simulink model "Lateral_control"  (R2022a)
settings: Solver=VariableStepAuto  StartTime=0.0  StopTime=15  RelTol=1e-3
values from neighbouring files (symbols this model uses):
  Cf = 19000    [main.m]
  Cr = 33000    [main.m]
  Iz = 2875    [main.m]
  Kfb = K(1,1:end-2)    [main.m]
  Kff = K(1,5:end)    [main.m]
  Lf = 1.2    [main.m]
  Lr = 1.6    [main.m]
  m = 1575    [main.m]
  Vx = 10    [main.m]
  x_0 = [0 0 0 0]'    [main.m]
undefined symbols (not defined in the file or in its folder): driving, sigbuilder_block
libraries: drivingscenarioandsensors x2
settings Model: Creator=User  LastModifiedBy=User

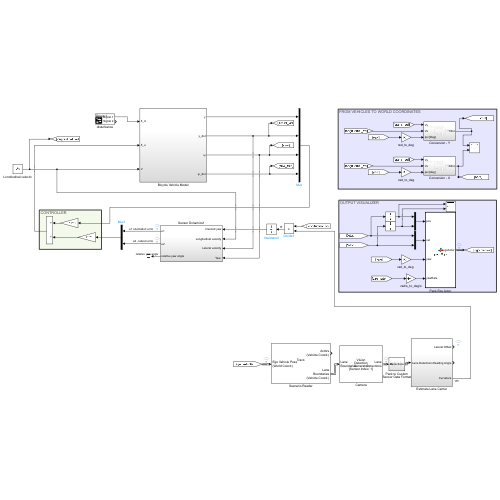
[thumbnail: Simulink's stored preview of the top-level diagram]
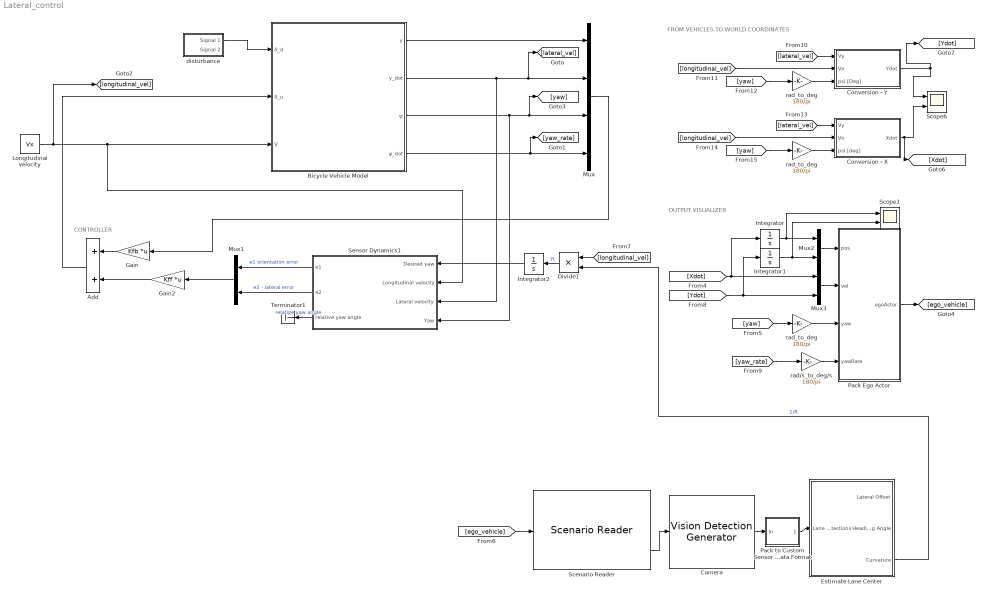
== system Lateral_control ==
  note: CONTROLLER
  note: FROM VEHICLES TO WORLD COORDINATES
  note: OUTPUT VISUALIZER
  Add : Sum
  Bicycle Vehicle Model : Subsystem
  Camera : drivingscenarioandsensors/Vision Detection Generator  SensorIndex=1  DetectorOutput=Lanes only  UpdateInterval=0.01  LaneUpdateInterval=0.01  SensorLocation=[1.9 0]  Height=1.1  Yaw=0  Pitch=1  Roll=0  BusNameSource=Auto  BusName=BusObjectDetections  BusName2Source=Property  BusName2=BusVision  MaxNumDetectionsSource=Property  MaxNumDetections=50  MaxNumLanesSource=Property  MaxNumLanes=2  DetectionCoordinates=Ego Cartesian  SimulateUsing=Interpreted execution  MaxRange=150  BoundingBoxAccuracy=5  ProcessNoiseIntensity=5  MaxSpeed=50  MaxAllowedOcclusion=0.5  MinObjectImageSize=[15 15]  DetectionProbability=0.9  FalsePositivesPerImage=0.1  MinLaneImageSize=[20 3]  LaneBoundaryAccuracy=3  HasNoise=on  InitialSeedSource=Repeatable  InitialSeed=0  UsedSeed=0  ActorProfilesSource=Parameters  ActorProfilesParameters=driving.internal.ActorProfilesParameters  ActorProfilesExpression=[struct('ActorID',1,'ClassID',1,'Length',4.7,'Width',1.8,'Height',1.4,'OriginOffset',[-1.35 0 0],'MeshVertices',[3.7 -0.9 1.4;3.7 0.9 1.4;-1 0.9 1.4;-1 -0.9 1.4;3.7 -0.9 0;3.7 0.9 0;-1 0.9 0;-1 -0.9 0],'MeshFaces',[6 2 1;1 5 6;8 4 3;3 7 8;6 7 3;3 2 6;5 1 4;4 8 5;4 1 2;2 3 4;7 6 5;5 8 7],'RCSPattern',[10 10;10 10],'RCSAzimuthAngles',[-180 180],'RCSElevationAngles',[-90 90])]  Intrinsics=driving.internal.cameraIntrinsics('FocalLength',[800 800],'PrincipalPoint',[320 240],'ImageSize',[480 640],'RadialDistortion',[0 0],'TangentialDistortion',[0 0],'Skew',0)
  Conversion - X : Subsystem
  Conversion - Y : Subsystem
  Divide1 : Product  Inputs=**
  Estimate Lane Center : Subsystem  VariantControl=v2
  Gain : Gain  Gain=Kfb  Multiplication=Matrix(K*u)
  Gain2 : Gain  Gain=Kff  Multiplication=Matrix(K*u)
  Integrator : Integrator  InitialCondition=1.64
  Integrator1 : Integrator  InitialCondition=0.05
  Integrator2 : Integrator
  Longitudinal velocity : Constant  Value=Vx  SampleTime=-1
  Mux : Mux
  Mux1 : Mux  Inputs=2
  Mux2 : Mux  Inputs=2
  Mux3 : Mux  Inputs=2
  Pack Ego Actor : MATLAB Function  TreatAsAtomicUnit=on
  Pack to Custom Sensor Data Format : Subsystem
  Scenario Reader : drivingscenarioandsensors/Scenario Reader  ScenarioSource=From file  ScenarioFileName=Track.mat  ScenarioVariableName=scenario  OutputCoordinateSystem=Vehicle coordinates  EgoVehicleSource=Input port  EgoVehicleActorID=1  OrientVehiclesOnRoad=off  OutputEgoVehiclePose=off  OutputEgoVehicleState=off  SampleTime=0.01  LaneBoundaryOutput=Ego vehicle lane boundaries  LaneBoundaryDistance=linspace(-150, 150, 101)  LaneBoundaryLocation=Center of lane markings  BusNameSource=Auto  BusName=BusActors  BusNumActorsSource=Scenario  BusNumActors=100  BusName2Source=Auto  BusName2=BusLaneBoundaries  BusNumLaneBoundariesSource=Scenario  BusNumLaneBoundaries=10  BusName3Source=Auto  BusName3=BusEgoActor  BusName4Source=Auto  BusName4=BusEgoState  ShowCoordinateLabels=on  SimulateUsing=Interpreted execution
  Scope1 : Scope  NumInputPorts=2
  Scope6 : Scope  NumInputPorts=2
  Sensor Dynamics1 : Subsystem
  Terminator1 : Terminator
  disturbance : Subsystem  Tag=STV Subsys  LoadFcn=sigbuilder_block('load');  StartFcn=sigbuilder_block('start');  StopFcn=sigbuilder_block('stop');  ClipboardFcn=sigbuilder_block('clipboard');  mask(Sigbuilder block){tuvar=[0:10]}
      mask help: Simulink:masks:SigbuilderBlock_MD
      mask init:
      | if ~strcmp(get_param(bdroot(gcbh),'SimulationStatus'),'stopped') tuvar = sigbuilder_block('maskInit'); end
      settings: CopyFcn=sigbuilder_block('copy');  DeleteFcn=sigbuilder_block('delete');  ModelCloseFcn=sigbuilder_block('modelClose');  PreSaveFcn=sigbuilder_block('preSave');  PauseFcn=sigbuilder_block('pause');  ContinueFcn=sigbuilder_block('continue');  NameChangeFcn=sigbuilder_block('namechange');  OpenFcn=sigbuilder_block('open',[5.4 44.4 1141.2 541.8 ]);  CloseFcn=sigbuilder_block('close');
      mask Display: plot(0, 0, 100, 100,[2, 2, 32, 32, 2], [68, 8, 8, 68, 68],[32, 2], [38, 38], [32, 19, 2],[53, 60, 44], [32, 17, 17, 2],[16, 16, 31, 31]);txt = getActiveGroup(gcbh);text(2, 100, txt,'verticalAlignment', 'top');
  rad/s_to_deg/s : Gain  Gain=180/pi
  rad_to_deg : Gain  Gain=180/pi
  "rad_to_deg " : Gain  Gain=180/pi
  "rad_to_deg  " : Gain  Gain=180/pi
  wires:
  Add/1 -> Bicycle Vehicle Model/2(δ_u)
  rad_to_deg/1 -> Conversion - X/3(psi [deg])
  [longitudinal_vel] -> Conversion - X/2(Vx)
  Bicycle Vehicle Model/4(ψ_dot) -> [yaw_rate], Mux/4
  Pack to Custom Sensor Data Format/1(Lane Detections) -> Estimate Lane Center/1(Lane Detections)
  Conversion - Y/1(Ydot) -> [Ydot], Scope6/1
  Divide1/1 -> Integrator2/1  "R"
  "rad_to_deg "/1 -> Conversion - Y/3(psi [Deg])
  Integrator/1 -> Scope1/1, Mux2/1
  rad/s_to_deg/s/1 -> Pack Ego Actor/4(yawRate)
  Mux1/1 -> Gain2/1
  [lateral_vel] -> Conversion - X/1(Vy)
  Integrator1/1 -> Scope1/2, Mux2/2
  Gain2/1 -> Add/2
  Mux2/1 -> Pack Ego Actor/1(pos)
  Mux3/1 -> Pack Ego Actor/2(vel)
  [yaw_rate] -> rad/s_to_deg/s/1
  Bicycle Vehicle Model/2(y_dot) -> Sensor Dynamics1/3(Lateral velocity), [lateral_vel], Mux/2
  "rad_to_deg  "/1 -> Pack Ego Actor/3(yaw)
  Sensor Dynamics1/1(e1) -> Mux1/1  "e1 orientation error"
  Camera/1 -> Pack to Custom Sensor Data Format/1(In)
  [yaw] -> "rad_to_deg  "/1
  Conversion - X/1(Xdot) -> Scope6/2, [Xdot]
  Sensor Dynamics1/2(e2) -> Mux1/2  "e2 - lateral error"
  Sensor Dynamics1/3(relative yaw angle) -> Terminator1/1  "relative yaw angle"
  Integrator2/1 -> Sensor Dynamics1/1(Desired yaw)
  [Ydot] -> Integrator1/1, Mux3/2
  [Xdot] -> Integrator/1, Mux3/1
  [yaw] -> "rad_to_deg "/1
  [ego_vehicle] -> Scenario Reader/1
  [longitudinal_vel] -> Conversion - Y/2(Vx)
  [longitudinal_vel] -> Divide1/1
  Pack Ego Actor/1(egoActor) -> [ego_vehicle]
  [lateral_vel] -> Conversion - Y/1(Vy)
  Bicycle Vehicle Model/3(ψ) -> Sensor Dynamics1/4("Yaw "), [yaw], Mux/3
  Gain/1 -> Add/1
  [yaw] -> rad_to_deg/1
  Scenario Reader/2 -> Camera/1
  Bicycle Vehicle Model/1(y) -> Mux/1
  Mux/1 -> Gain/1
  Longitudinal velocity/1 -> Sensor Dynamics1/2(Longitudinal velocity), Bicycle Vehicle Model/3(V), [longitudinal_vel]
  Estimate Lane Center/3(Curvature) -> Divide1/2  "1/R"
  disturbance/1(Signal 1) -> Bicycle Vehicle Model/1(δ_d)

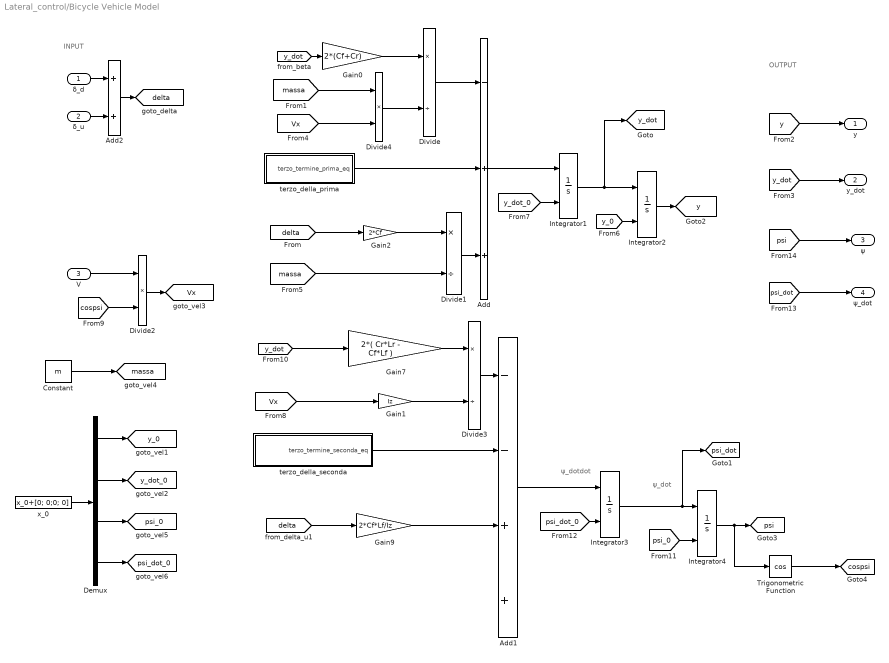
== system Lateral_control/Bicycle Vehicle Model ==
  note: ψ_dot
  note: OUTPUT
  note: INPUT
  note: ψ_dotdot
  δ_d : Inport
  δ_u : Inport  Port=2
  V : Inport  Port=3
  Add : Sum  Inputs=-++
  Add1 : Sum  Inputs=--++
  Add2 : Sum
  Constant : Constant  Value=m
  Demux : Demux
  Divide : Product  Inputs=*/
  Divide1 : Product  Inputs=*/
  Divide2 : Product  Inputs=**
  Divide3 : Product  Inputs=*/
  Divide4 : Product  Inputs=**
  Gain0 : Gain  Gain=2*(Cf+Cr)
  Gain1 : Gain  Gain=Iz
  Gain2 : Gain  Gain=2*Cf
  Gain7 : Gain  Gain="2*( Cr*Lr  - Cf*Lf )"
  Gain9 : Gain  Gain=2*Cf*Lf/Iz
  Integrator1 : Integrator  InitialConditionSource=external
  Integrator2 : Integrator  InitialConditionSource=external
  Integrator3 : Integrator  InitialConditionSource=external
  Integrator4 : Integrator  InitialConditionSource=external  LowerSaturationLimit=0
  Trigonometric Function : Trigonometry  Operator=cos
  terzo_della_prima : Subsystem
  terzo_della_seconda : Subsystem
  "x_0 " : Constant  Value=x_0+[0; 0;0; 0]
  y : Outport
  y_dot : Outport  Port=2
  ψ : Outport  Port=3
  ψ_dot : Outport  Port=4
  tag scope: Vx=global, cospsi=global, delta=global, massa=global, psi=global, psi_0=global, psi_dot=global, psi_dot_0=global, y=global, y_0=global, y_dot=global, y_dot_0=global
  wires:
  [psi] -> ψ/1
  [psi_dot] -> ψ_dot/1
  [psi_dot_0] -> Integrator3/2
  [psi_0] -> Integrator4/2
  [cospsi] -> Divide2/2
  Trigonometric Function/1 -> [cospsi]
  Divide2/1 -> [Vx]
  Integrator4/1 -> [psi], Trigonometric Function/1
  [Vx] -> Gain1/1
  Gain1/1 -> Divide3/2
  Divide3/1 -> Add1/1
  [y_0] -> Integrator2/2
  [y_dot_0] -> Integrator1/2
  Demux/4 -> [psi_dot_0]
  Demux/3 -> [psi_0]
  Integrator2/1 -> [y]
  Integrator1/1 -> [y_dot], Integrator2/1
  Divide1/1 -> Add/3
  [massa] -> Divide1/2
  Divide/1 -> Add/1
  [Vx] -> Divide4/2
  [massa] -> Divide4/1
  Divide4/1 -> Divide/2
  "x_0 "/1 -> Demux/1
  [delta] -> Gain2/1
  Add2/1 -> [delta]
  Gain9/1 -> Add1/3
  terzo_della_seconda/1("terzo_termine_seconda_eq ") -> Add1/2
  Gain2/1 -> Divide1/1
  terzo_della_prima/1("terzo_termine_prima_eq ") -> Add/2
  Demux/2 -> [y_dot_0]
  Demux/1 -> [y_0]
  Constant/1 -> [massa]
  Integrator3/1 -> Integrator4/1, [psi_dot]
  Add/1 -> Integrator1/1
  [y_dot] -> Gain7/1
  [y_dot] -> Gain0/1
  [y_dot] -> y_dot/1
  [y] -> y/1
  [delta] -> Gain9/1
  Gain7/1 -> Divide3/1
  Add1/1 -> Integrator3/1
  Gain0/1 -> Divide/1
  V/1 -> Divide2/1
  δ_u/1 -> Add2/2
  δ_d/1 -> Add2/1

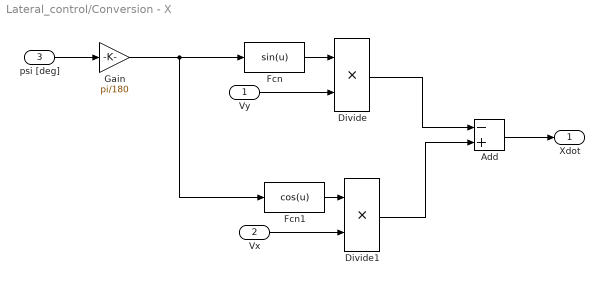
== system Lateral_control/Conversion - X ==
  Vy : Inport
  Vx : Inport  Port=2
  psi [deg] : Inport  Port=3
  Add : Sum  Inputs=-+
  Divide : Product  Inputs=**
  Divide1 : Product  Inputs=**
  Fcn : Fcn  Expr=sin(u)
  Fcn1 : Fcn  Expr=cos(u)
  Gain : Gain  Gain=pi/180
  Xdot : Outport
  wires:
  Gain/1 -> Fcn/1, Fcn1/1
  Add/1 -> Xdot/1
  Divide1/1 -> Add/2
  Vx/1 -> Divide1/2
  Fcn1/1 -> Divide1/1
  Divide/1 -> Add/1
  Vy/1 -> Divide/2
  Fcn/1 -> Divide/1
  psi [deg]/1 -> Gain/1

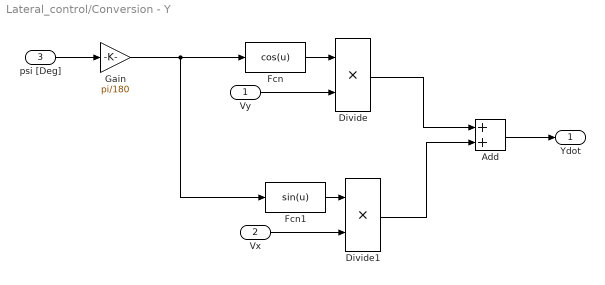
== system Lateral_control/Conversion - Y ==
  Vy : Inport
  Vx : Inport  Port=2
  psi [Deg] : Inport  Port=3
  Add : Sum
  Divide : Product  Inputs=**
  Divide1 : Product  Inputs=**
  Fcn : Fcn  Expr=cos(u)
  Fcn1 : Fcn  Expr=sin(u)
  Gain : Gain  Gain=pi/180
  Ydot : Outport
  wires:
  psi [Deg]/1 -> Gain/1
  Fcn/1 -> Divide/1
  Vy/1 -> Divide/2
  Divide/1 -> Add/1
  Fcn1/1 -> Divide1/1
  Vx/1 -> Divide1/2
  Divide1/1 -> Add/2
  Add/1 -> Ydot/1
  Gain/1 -> Fcn1/1, Fcn/1

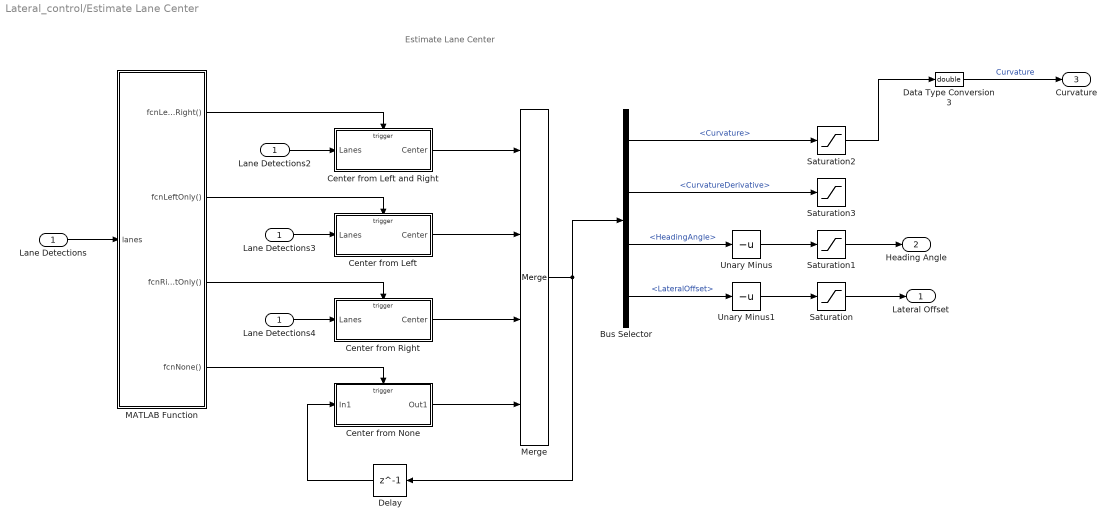
== system Lateral_control/Estimate Lane Center ==
  note: Estimate Lane Center
  Lane Detections : Inport
  Bus Selector : BusSelector  OutputSignals=Curvature,CurvatureDerivative,HeadingAngle,LateralOffset
  Center from Left : Subsystem  TreatAsAtomicUnit=on
  Center from Left and Right : Subsystem  TreatAsAtomicUnit=on
  Center from None : Subsystem  TreatAsAtomicUnit=on
  Center from Right : Subsystem  TreatAsAtomicUnit=on
  Data Type Conversion3 : DataTypeConversion  OutDataTypeStr=double  SaturateOnIntegerOverflow=off  RndMeth=Floor
  Delay : Delay  DelayLength=1
  Lane Detections2 : InportShadow
  Lane Detections3 : InportShadow
  Lane Detections4 : InportShadow
  MATLAB Function : MATLAB Function  TreatAsAtomicUnit=on
  Merge : Merge  Inputs=4
  Saturation : Saturate
  Saturation1 : Saturate  UpperLimit=0.6  LowerLimit=-0.6
  Saturation2 : Saturate  UpperLimit=0.15  LowerLimit=-0.15
  Saturation3 : Saturate  UpperLimit=0.15  LowerLimit=-0.15
  Unary Minus : UnaryMinus
  Unary Minus1 : UnaryMinus
  Lateral Offset : Outport  VectorParamsAs1DForOutWhenUnconnected=off
  Heading Angle : Outport  Port=2  VectorParamsAs1DForOutWhenUnconnected=off
  Curvature : Outport  Port=3  VectorParamsAs1DForOutWhenUnconnected=off
  wires:
  Center from Right/1(Center) -> Merge/3
  Lane Detections3/1 -> Center from Left/1(Lanes)
  Lane Detections4/1 -> Center from Right/1(Lanes)
  MATLAB Function/2(fcnLeftOnly()) -> Center from Left/Trigger
  Center from None/1(Out1) -> Merge/4
  MATLAB Function/1(fcnLeftAndRight()) -> Center from Left and Right/Trigger
  Delay/1 -> Center from None/1(In1)
  Center from Left and Right/1(Center) -> Merge/1
  Lane Detections/1 -> MATLAB Function/1(lanes)
  Lane Detections2/1 -> Center from Left and Right/1(Lanes)
  MATLAB Function/3(fcnRightOnly()) -> Center from Right/Trigger
  MATLAB Function/4(fcnNone()) -> Center from None/Trigger
  Center from Left/1(Center) -> Merge/2
  Merge/1 -> Bus Selector/1, Delay/1
  Saturation2/1 -> Data Type Conversion3/1
  Saturation1/1 -> Heading Angle/1
  Saturation/1 -> Lateral Offset/1
  Unary Minus/1 -> Saturation1/1
  Bus Selector/2 -> Saturation3/1  "<CurvatureDerivative>"
  Bus Selector/1 -> Saturation2/1  "<Curvature>"
  Unary Minus1/1 -> Saturation/1
  Bus Selector/4 -> Unary Minus1/1  "<LateralOffset>"
  Bus Selector/3 -> Unary Minus/1  "<HeadingAngle>"
  Data Type Conversion3/1 -> Curvature/1  "Curvature"

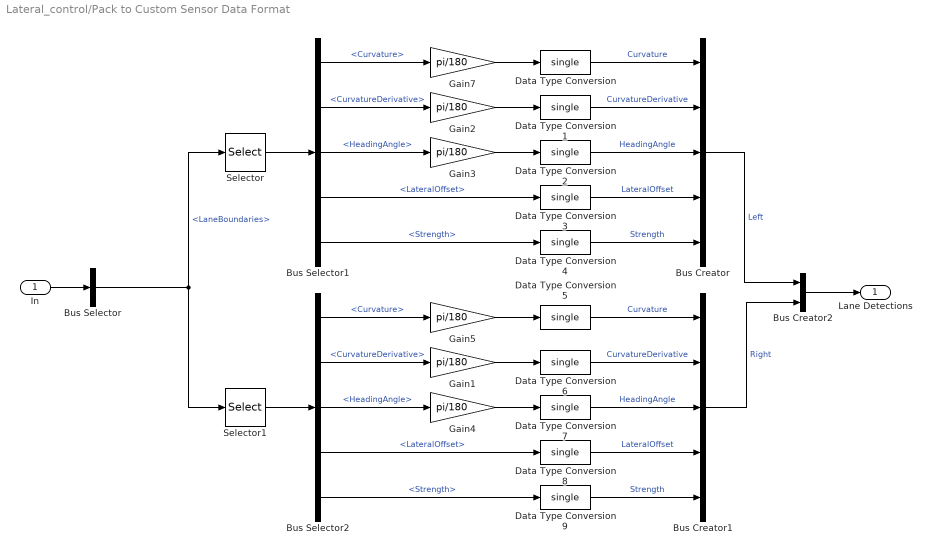
== system Lateral_control/Pack to Custom Sensor Data Format ==
  In : Inport
  Bus Creator : BusCreator  Inputs=5  OutDataTypeStr=Bus: LaneSensorBoundaries
  Bus Creator1 : BusCreator  Inputs=5  OutDataTypeStr=Bus: LaneSensorBoundaries
  Bus Creator2 : BusCreator  Inputs=2  OutDataTypeStr=Bus: LaneSensor
  Bus Selector : BusSelector  OutputSignals=LaneBoundaries
  Bus Selector1 : BusSelector  OutputSignals=Curvature,CurvatureDerivative,HeadingAngle,LateralOffset,Strength
  Bus Selector2 : BusSelector  OutputSignals=Curvature,CurvatureDerivative,HeadingAngle,LateralOffset,Strength
  Data Type Conversion{,1..9} (10 alike) : DataTypeConversion  OutDataTypeStr=single  SaturateOnIntegerOverflow=off  RndMeth=Floor
  Gain{1..5,7} (6 alike) : Gain  Gain=pi/180
  Selector : Selector  InputPortWidth=2  IndexOptions=Index vector (dialog)  Indices=1  OutputSizes=1
  Selector1 : Selector  InputPortWidth=2  IndexOptions=Index vector (dialog)  Indices=2  OutputSizes=1
  Lane Detections : Outport  VectorParamsAs1DForOutWhenUnconnected=off
  wires:
  In/1 -> Bus Selector/1
  Bus Selector/1 -> Selector/1, Selector1/1  "<LaneBoundaries>"
  Selector/1 -> Bus Selector1/1
  Bus Selector1/2 -> Gain2/1  "<CurvatureDerivative>"
  Bus Selector1/1 -> Gain7/1  "<Curvature>"
  Bus Selector1/3 -> Gain3/1  "<HeadingAngle>"
  Gain7/1 -> Data Type Conversion/1
  Gain2/1 -> Data Type Conversion1/1
  Gain3/1 -> Data Type Conversion2/1
  Bus Selector1/4 -> Data Type Conversion3/1  "<LateralOffset>"
  Bus Selector1/5 -> Data Type Conversion4/1  "<Strength>"
  Data Type Conversion/1 -> Bus Creator/1  "Curvature"
  Data Type Conversion1/1 -> Bus Creator/2  "CurvatureDerivative"
  Data Type Conversion2/1 -> Bus Creator/3  "HeadingAngle"
  Data Type Conversion3/1 -> Bus Creator/4  "LateralOffset"
  Data Type Conversion4/1 -> Bus Creator/5  "Strength"
  Data Type Conversion9/1 -> Bus Creator1/5  "Strength"
  Data Type Conversion6/1 -> Bus Creator1/2  "CurvatureDerivative"
  Data Type Conversion7/1 -> Bus Creator1/3  "HeadingAngle"
  Data Type Conversion8/1 -> Bus Creator1/4  "LateralOffset"
  Data Type Conversion5/1 -> Bus Creator1/1  "Curvature"
  Bus Selector2/1 -> Gain5/1  "<Curvature>"
  Selector1/1 -> Bus Selector2/1
  Bus Selector2/4 -> Data Type Conversion8/1  "<LateralOffset>"
  Bus Selector2/5 -> Data Type Conversion9/1  "<Strength>"
  Bus Selector2/2 -> Gain1/1  "<CurvatureDerivative>"
  Gain4/1 -> Data Type Conversion7/1
  Gain5/1 -> Data Type Conversion5/1
  Gain1/1 -> Data Type Conversion6/1
  Bus Selector2/3 -> Gain4/1  "<HeadingAngle>"
  Bus Creator2/1 -> Lane Detections/1
  Bus Creator/1 -> Bus Creator2/1  "Left"
  Bus Creator1/1 -> Bus Creator2/2  "Right"

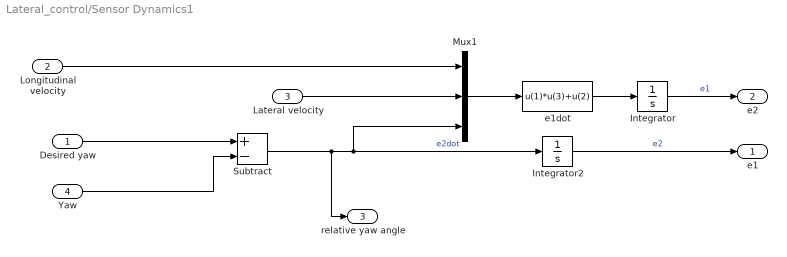
== system Lateral_control/Sensor Dynamics1 ==
  Desired yaw : Inport
  Longitudinal velocity : Inport  Port=2
  Lateral velocity : Inport  Port=3
  "Yaw " : Inport  Port=4
  Integrator : Integrator
  Integrator2 : Integrator
  Mux1 : Mux  Inputs=[1 1 1]
  Subtract : Sum  Inputs=+-
  e1dot : Fcn  Expr=u(1)*u(3)+u(2)
  e1 : Outport  VectorParamsAs1DForOutWhenUnconnected=off
  e2 : Outport  Port=2  VectorParamsAs1DForOutWhenUnconnected=off
  relative yaw angle : Outport  Port=3  VectorParamsAs1DForOutWhenUnconnected=off
  wires:
  Integrator2/1 -> e1/1  "e2"
  Mux1/1 -> e1dot/1
  e1dot/1 -> Integrator/1
  Longitudinal velocity/1 -> Mux1/1
  Lateral velocity/1 -> Mux1/2
  Integrator/1 -> e2/1  "e1"
  Desired yaw/1 -> Subtract/1
  "Yaw "/1 -> Subtract/2
  Subtract/1 -> relative yaw angle/1, Mux1/3, Integrator2/1  "e2dot"

== system Lateral_control/disturbance ==
  Demux : Demux  Tag=STV Demux  Outputs=2
      settings: DisplayOption=none
  FromWs : FromWorkspace  Tag=STV FromWs  VariableName=tuvar
      SigBuilderData=|
      | common.afterFinalStr = 'Extrapolate'
      | common.sampleTime = 0
      | dataSet.timeRange = [0 50]
      | dataSet.name = 'Group 1'
      | sbobj.Groups.Name = 'Group 1'
      | sbobj.Groups.Signals(1).Name = 'Signal 1'
      | sbobj.Groups.Signals(1).XData = [0 0.105263157895 0.210526315789 0.315789473684 0.421052631579 0.526315789474 0.631578947368 0.736842105263 0.842105263158 0.947368421053 1.05263157895 1.15789473684 1.26315789474 1.36842105263 1.47368421053 1.57894736842 1.68421052632 1.78947368421 1.89473684211 2 2.10526315789 2.21052631579 2.31578947368 2.42105263158 2.52631578947 2.63157894737 2.73684210526 2.84210526316 2.94736842105 3.05263157895 3.15789473684 3.26315789474 3.36842105263 3.47368421053 3.57894736842 3.68421052632 3.78947368421 3.89473684211 4 4.10526315789 4.21052631579 4.31578947368 4.42105263158 4.52631578947 4.63157894737 4.73684210526 4.84210526316 4.94736842105 5.05263157895 5.15789473684 5.26315789474 5.36842105263 5.47368421053 5.57894736842 5.68421052632 5.78947368421 5.89473684211 6 6.10526315789 6.21052631579 6.31578947368 6.42105263158 6.52631578947 6.63157894737 6.73684210526 6.84210526316 6.94736842105 7.05263157895 7.15789473684 7.26315789474 7.36842105263 7.47368421053 7.57894736842 50]
      | sbobj.Groups.Signals(1).YData = [0 0 0 0 0 0 0 0 0 0 0 0 0 0 0 0 0 0 0 0 0 0 0 0 0 0 0 0 0 0 0 0 0 0 0 0 0 0 0 0.324699469205 0.61421271269 0.837166478263 0.969400265939 0.996584493007 0.915773326655 0.735723910673 0.475947393037 0.13 -0.164594590281 -0.475947393037 -0.735723910673 -0.915773326655 -0.996584493007 -0.969400265939 -0.837166478263 -0.61421271269 -0.324699469205 0 0 0 0 0 0 0 0 0 0 0 0 0 0 0 0 0]
      | sbobj.Groups.Signals(2).Name = 'Signal 2'
      | sbobj.Groups.Signals(2).XData = [0 15.35 15.35 30 30 50]
      | sbobj.Groups.Signals(2).YData = [0 0 1 1 0 0]
      | sbobj.Groups.TimeRange = [0 50]
  Signal 1 : Outport  Tag=STV Outport
  Signal 2 : Outport  Tag=STV Outport  Port=2
  wires:
  Demux/1 -> Signal 1/1
  FromWs/1 -> Demux/1
  Demux/2 -> Signal 2/1

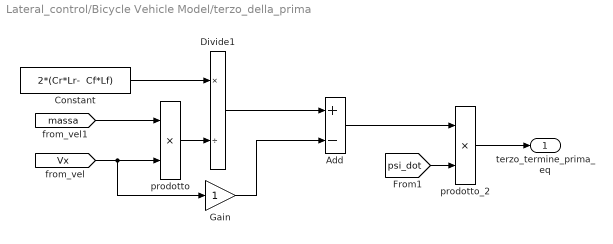
== system Lateral_control/Bicycle Vehicle Model/terzo_della_prima ==
  Add : Sum  Inputs=+-
  Constant : Constant  Value="2*(Cr*Lr-  Cf*Lf)"
  Divide1 : Product  Inputs=*/
  Gain : Gain
  prodotto : Product  Inputs=**
  prodotto_2 : Product  Inputs=**
  "terzo_termine_prima_eq " : Outport
  wires:
  Gain/1 -> Add/2
  [massa] -> prodotto/1
  prodotto/1 -> Divide1/2
  Add/1 -> prodotto_2/1
  [Vx] -> prodotto/2, Gain/1
  prodotto_2/1 -> "terzo_termine_prima_eq "/1
  [psi_dot] -> prodotto_2/2
  Divide1/1 -> Add/1
  Constant/1 -> Divide1/1

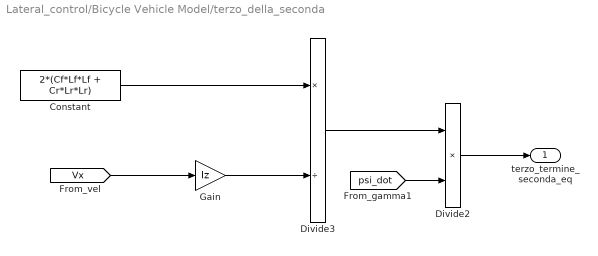
== system Lateral_control/Bicycle Vehicle Model/terzo_della_seconda ==
  Constant : Constant  Value=2*(Cf*Lf*Lf + Cr*Lr*Lr)
  Divide2 : Product  Inputs=**
  Divide3 : Product  Inputs=*/
  Gain : Gain  Gain=Iz
  "terzo_termine_seconda_eq " : Outport
  wires:
  Divide2/1 -> "terzo_termine_seconda_eq "/1
  [psi_dot] -> Divide2/2
  Gain/1 -> Divide3/2
  [Vx] -> Gain/1
  Divide3/1 -> Divide2/1
  Constant/1 -> Divide3/1

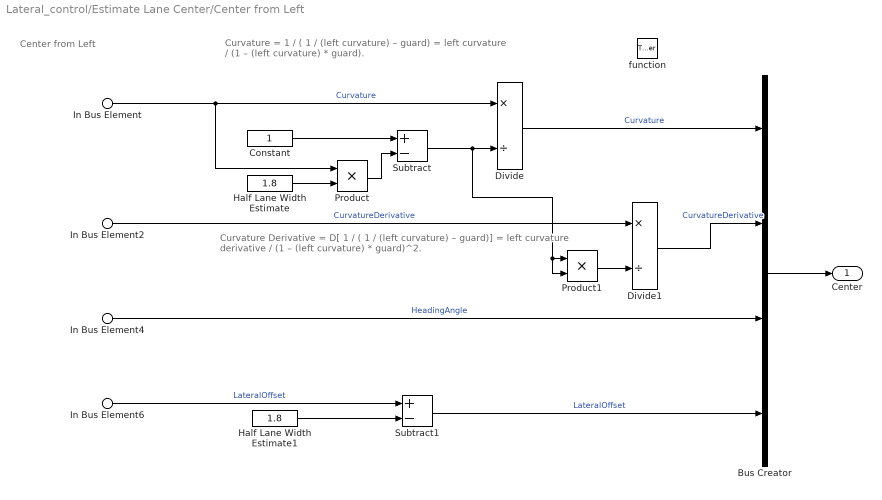
== system Lateral_control/Estimate Lane Center/Center from Left ==
  note: Curvature Derivative
      | = D[ 1 / ( 1 / (left curvature) – guard)]
      | = left curvature derivative / (1 – (left curvature) * guard)^2.
  note: Center from Left
  note: Curvature
      | = 1 / ( 1 / (left curvature) – guard)
      | = left curvature / (1 – (left curvature) * guard).
  In Bus Element : Inport  PortName=Lanes  Element=Left.Curvature
  In Bus Element2 : Inport  PortName=Lanes  Element=Left.CurvatureDerivative
  In Bus Element4 : Inport  PortName=Lanes  Element=Left.HeadingAngle
  In Bus Element6 : Inport  PortName=Lanes  Element=Left.LateralOffset
  function : TriggerPort  TriggerType=function-call  VariantControl=Variant
  Bus Creator : BusCreator  Inputs=4
  Constant : Constant  OutDataTypeStr=Inherit: Inherit via back propagation
  Divide : Product  Inputs=*/
  Divide1 : Product  Inputs=*/
  Half Lane Width Estimate : Constant  Value=1.8  OutDataTypeStr=Inherit: Inherit via back propagation
  Half Lane Width Estimate1 : Constant  Value=1.8  OutDataTypeStr=Inherit: Inherit via back propagation
  Product : Product
  Product1 : Product
  Subtract : Sum  Inputs=+-
  Subtract1 : Sum  Inputs=+-
  Center : Outport  VectorParamsAs1DForOutWhenUnconnected=off
  wires:
  Product/1 -> Subtract/2
  Half Lane Width Estimate1/1 -> Subtract1/2
  In Bus Element6/1 -> Subtract1/1  "LateralOffset"
  Product1/1 -> Divide1/2
  In Bus Element2/1 -> Divide1/1  "CurvatureDerivative"
  Constant/1 -> Subtract/1
  Half Lane Width Estimate/1 -> Product/2
  Subtract/1 -> Divide/2, Product1/1, Product1/2
  In Bus Element/1 -> Divide/1, Product/1  "Curvature"
  Subtract1/1 -> Bus Creator/4  "LateralOffset"
  In Bus Element4/1 -> Bus Creator/3  "HeadingAngle"
  Divide/1 -> Bus Creator/1  "Curvature"
  Divide1/1 -> Bus Creator/2  "CurvatureDerivative"
  Bus Creator/1 -> Center/1

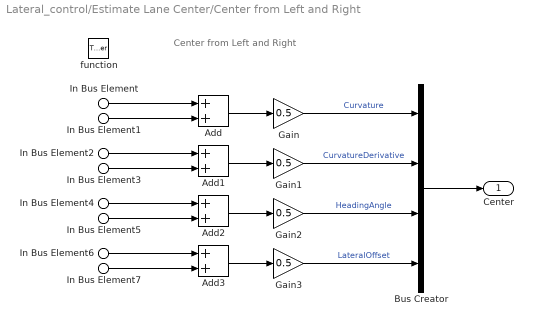
== system Lateral_control/Estimate Lane Center/Center from Left and Right ==
  note: Center from Left and Right
  In Bus Element : Inport  PortName=Lanes  Element=Left.Curvature
  In Bus Element2 : Inport  PortName=Lanes  Element=Left.CurvatureDerivative
  In Bus Element4 : Inport  PortName=Lanes  Element=Left.HeadingAngle
  In Bus Element6 : Inport  PortName=Lanes  Element=Left.LateralOffset
  In Bus Element1 : Inport  PortName=Lanes  Element=Right.Curvature
  In Bus Element3 : Inport  PortName=Lanes  Element=Right.CurvatureDerivative
  In Bus Element5 : Inport  PortName=Lanes  Element=Right.HeadingAngle
  In Bus Element7 : Inport  PortName=Lanes  Element=Right.LateralOffset
  function : TriggerPort  TriggerType=function-call  VariantControl=Variant
  Add{,1..3} (4 alike) : Sum
  Bus Creator : BusCreator  Inputs=4
  Gain{,1..3} (4 alike) : Gain  Gain=0.5
  Center : Outport  VectorParamsAs1DForOutWhenUnconnected=off
  wires:
  In Bus Element6/1 -> Add3/1
  In Bus Element7/1 -> Add3/2
  In Bus Element5/1 -> Add2/2
  In Bus Element4/1 -> Add2/1
  In Bus Element3/1 -> Add1/2
  In Bus Element2/1 -> Add1/1
  In Bus Element1/1 -> Add/2
  In Bus Element/1 -> Add/1
  Bus Creator/1 -> Center/1
  Gain3/1 -> Bus Creator/4  "LateralOffset"
  Add3/1 -> Gain3/1
  Gain2/1 -> Bus Creator/3  "HeadingAngle"
  Add2/1 -> Gain2/1
  Gain1/1 -> Bus Creator/2  "CurvatureDerivative"
  Add1/1 -> Gain1/1
  Gain/1 -> Bus Creator/1  "Curvature"
  Add/1 -> Gain/1

== system Lateral_control/Estimate Lane Center/Center from None ==
  In1 : Inport
  function : TriggerPort  TriggerType=function-call  VariantControl=Variant
  Out1 : Outport  VectorParamsAs1DForOutWhenUnconnected=off
  wires:
  In1/1 -> Out1/1

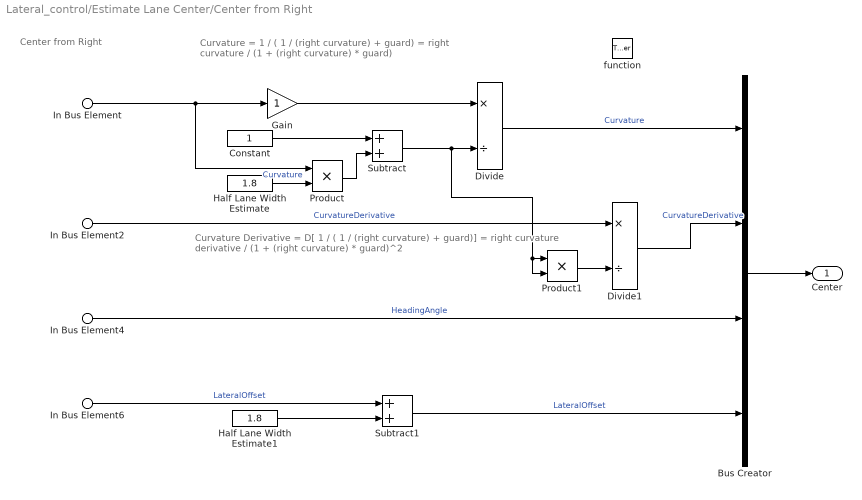
== system Lateral_control/Estimate Lane Center/Center from Right ==
  note: Curvature Derivative
      | = D[ 1 / ( 1 / (right curvature) + guard)]
      | = right curvature derivative / (1 + (right curvature) * guard)^2
  note: Curvature
      | = 1 / ( 1 / (right curvature) + guard)
      | = right curvature / (1 + (right curvature) * guard)
  note: Center from Right
  In Bus Element : Inport  PortName=Lanes  Element=Right.Curvature
  In Bus Element2 : Inport  PortName=Lanes  Element=Right.CurvatureDerivative
  In Bus Element4 : Inport  PortName=Lanes  Element=Right.HeadingAngle
  In Bus Element6 : Inport  PortName=Lanes  Element=Right.LateralOffset
  function : TriggerPort  TriggerType=function-call  VariantControl=Variant
  Bus Creator : BusCreator  Inputs=4
  Constant : Constant  OutDataTypeStr=Inherit: Inherit via back propagation
  Divide : Product  Inputs=*/
  Divide1 : Product  Inputs=*/
  Gain : Gain
  Half Lane Width Estimate : Constant  Value=1.8  OutDataTypeStr=Inherit: Inherit via back propagation
  Half Lane Width Estimate1 : Constant  Value=1.8  OutDataTypeStr=Inherit: Inherit via back propagation
  Product : Product
  Product1 : Product
  Subtract : Sum
  Subtract1 : Sum
  Center : Outport  VectorParamsAs1DForOutWhenUnconnected=off
  wires:
  Half Lane Width Estimate/1 -> Product/2
  Product/1 -> Subtract/2
  Constant/1 -> Subtract/1
  Subtract/1 -> Divide/2, Product1/1, Product1/2
  In Bus Element/1 -> Gain/1, Product/1  "Curvature"
  Bus Creator/1 -> Center/1
  Subtract1/1 -> Bus Creator/4  "LateralOffset"
  Divide/1 -> Bus Creator/1  "Curvature"
  In Bus Element6/1 -> Subtract1/1  "LateralOffset"
  Half Lane Width Estimate1/1 -> Subtract1/2
  In Bus Element4/1 -> Bus Creator/3  "HeadingAngle"
  Product1/1 -> Divide1/2
  Divide1/1 -> Bus Creator/2  "CurvatureDerivative"
  In Bus Element2/1 -> Divide1/1  "CurvatureDerivative"
  Gain/1 -> Divide/1

== matlab function Lateral_control/Pack Ego Actor ==
  data: pos input; egoActor output Bus: BusActors1Actors size=1; vel input; yaw input; yawRate input
function egoActor = packEgo(pos,vel,yaw,yawRate)
% Pack ego information into a single ego actor bus
%
% Imoprtant note:
% Output is a bus of type BusActorsActors. This is the same bus used by the
% Scenario Reader to output an individual actor. If you change the
% output bus name of Scenario Reader, change the output bus name here
% as well by clicking on 'Edit Data' in the menu above.

%Position x,y,z
%Velocity x,y,z
%Angular velocity wx, wy, wz

egoActor = struct(...
    'ActorID',1,...
    'Position', [pos(1) pos(2) 0], ...
    'Velocity', [vel(1) vel(2) 0], ...
    'Roll', 0, ...
    'Pitch', 0, ...
    'Yaw', yaw, ...
    'AngularVelocity', [0 0 yawRate]);

== matlab function Lateral_control/Estimate Lane Center/MATLAB Function ==
  data: lanes input
  events: fcnLeftAndRight output FUNCTION_CALL_EVENT; fcnLeftOnly output FUNCTION_CALL_EVENT; fcnRightOnly output FUNCTION_CALL_EVENT; fcnNone output FUNCTION_CALL_EVENT
function fcn(lanes)

leftStrength  = lanes.Left.Strength;
rightStrength = lanes.Right.Strength;

if (leftStrength > 0) && (rightStrength > 0)
   fcnLeftAndRight();
   
elseif leftStrength > 0
    fcnLeftOnly();
    
elseif rightStrength > 0
    fcnRightOnly();
    
else
    fcnNone();
end
